simulink model "osss"  (R2024b)
settings: Solver=VariableStepAuto  StartTime=0.0  StopTime=100  RelTol=1e-3
values from neighbouring files (symbols this model uses):
  A4 = horzcat([0;0;0;0], A4)    [stabilita_AS.m]
  BB = [0; B]    [stabilita_AS.m]
settings Model: Creator=costa  LastModifiedBy=costa

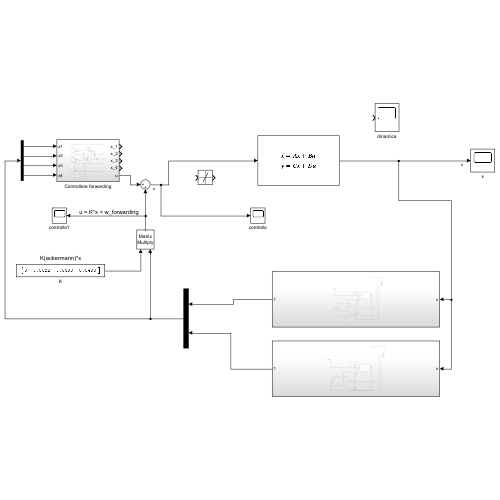
[thumbnail: Simulink's stored preview of the top-level diagram]
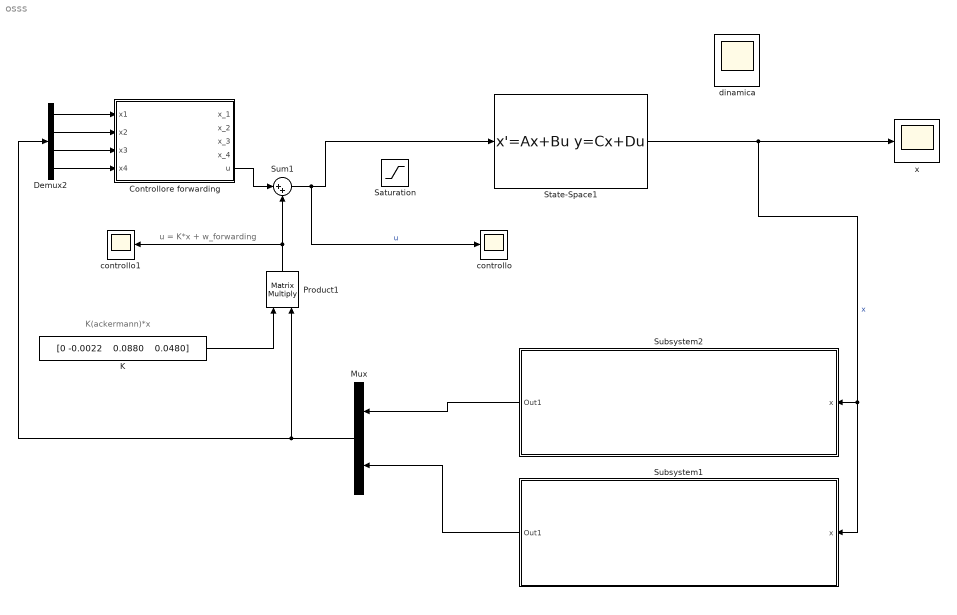
== system osss ==
  note: K(ackermann)*x
  note: u = K*x + w_forwarding
  Controllore forwarding : Subsystem
  Demux2 : Demux
  K : Constant  Value="[0 -0.0022    0.0880    0.0480]"  VectorParams1D=off
  Mux : Mux  Inputs=2
  Product1 : Product  Multiplication=Matrix(*)
  Saturation : Saturate
  State-Space1 : StateSpace  A=A4  B=BB  C=eye(4)  D=[0; 0; 0; 0]  InitialCondition=[1 1 1 1]
  Subsystem1 : Subsystem
  Subsystem2 : Subsystem
  Sum1 : Sum  Inputs=|++
  controllo : Scope
  controllo1 : Scope
  dinamica : Scope
  x : Scope
  wires:
  K/1 -> Product1/1
  Sum1/1 -> State-Space1/1, controllo/1  "u"
  Product1/1 -> controllo1/1, Sum1/2
  State-Space1/1 -> Subsystem2/1(x), Subsystem1/1(x), x/1  "x"
  Demux2/4 -> Controllore forwarding/4(x4)
  Demux2/3 -> Controllore forwarding/3(x3)
  Demux2/1 -> Controllore forwarding/1(x1)
  Demux2/2 -> Controllore forwarding/2(x2)
  Controllore forwarding/5(u) -> Sum1/1
  Mux/1 -> Demux2/1, Product1/2
  Subsystem1/1(Out1) -> Mux/2
  Subsystem2/1(Out1) -> Mux/1

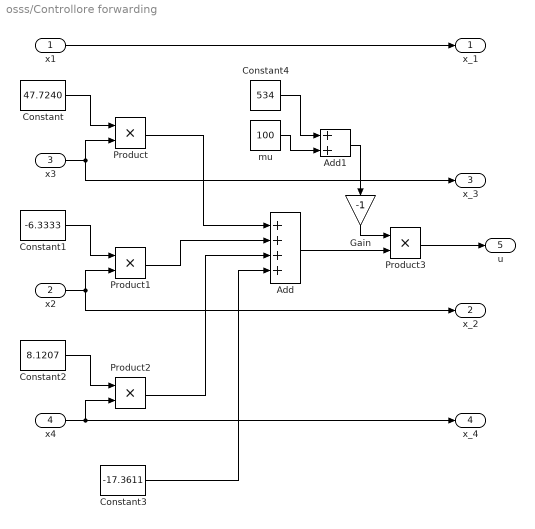
== system osss/Controllore forwarding ==
  x1 : Inport
  x2 : Inport  Port=2
  x3 : Inport  Port=3
  x4 : Inport  Port=4
  Add : Sum  Inputs=++++
  Add1 : Sum
  Constant : Constant  Value=47.7240
  Constant1 : Constant  Value=-6.3333
  Constant2 : Constant  Value=8.1207
  Constant3 : Constant  Value=-17.3611
  Constant4 : Constant  Value=534
  Gain : Gain  Gain=-1
  Product{,1..3} (4 alike) : Product
  mu : Constant  Value=100
  x_1 : Outport
  x_2 : Outport  Port=2
  x_3 : Outport  Port=3
  x_4 : Outport  Port=4
  u : Outport  Port=5
  wires:
  x3/1 -> x_3/1, Product/2
  Constant/1 -> Product/1
  Constant1/1 -> Product1/1
  x2/1 -> Product1/2, x_2/1
  Constant2/1 -> Product2/1
  x4/1 -> x_4/1, Product2/2
  Product/1 -> Add/1
  Product1/1 -> Add/2
  Product2/1 -> Add/3
  Constant3/1 -> Add/4
  Add/1 -> Product3/2
  Product3/1 -> u/1
  x1/1 -> x_1/1
  Constant4/1 -> Add1/1
  mu/1 -> Add1/2
  Add1/1 -> Gain/1
  Gain/1 -> Product3/1

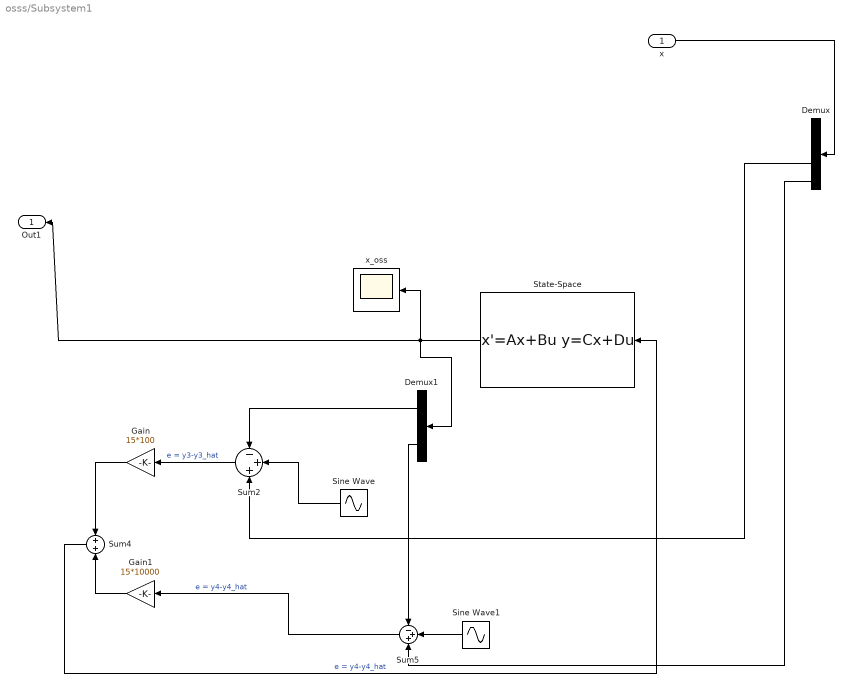
== system osss/Subsystem1 ==
  x : Inport
  Demux : Demux
  Demux1 : Demux  Outputs=2
  Gain : Gain  Gain=15*100
  Gain1 : Gain  Gain=15*10000
  Sine Wave : Sin  Amplitude=0.1  Frequency=2*pi*50  SampleTime=0
  Sine Wave1 : Sin  Amplitude=0.1  Frequency=2*pi*50  SampleTime=0
  State-Space : StateSpace  A=A4  B=BB  C=[0 0 1 0; 0 0 0 1]  D=[0; 0]  InitialCondition=[1 1 1 1]
  Sum2 : Sum  Inputs=-++
  Sum4 : Sum
  Sum5 : Sum  Inputs=-++
  x_oss : Scope
  Out1 : Outport
  wires:
  Gain1/1 -> Sum4/2
  State-Space/1 -> x_oss/1, Out1/1, Demux1/1
  x/1 -> Demux/1
  Sum5/1 -> Gain1/1  "e = y4-y4_hat"
  Sum2/1 -> Gain/1  "e = y3-y3_hat"
  Sine Wave1/1 -> Sum5/2
  Demux1/1 -> Sum2/1
  Demux/4 -> Sum5/3
  Sine Wave/1 -> Sum2/2
  Demux1/2 -> Sum5/1
  Sum4/1 -> State-Space/1  "e = y4-y4_hat"
  Demux/3 -> Sum2/3
  Gain/1 -> Sum4/1

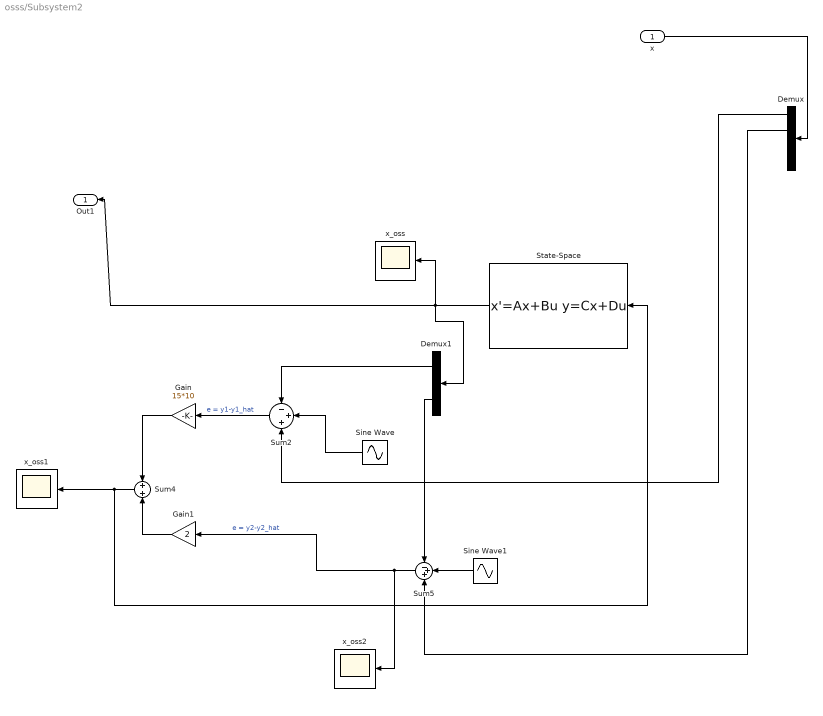
== system osss/Subsystem2 ==
  x : Inport
  Demux : Demux
  Demux1 : Demux  Outputs=2
  Gain : Gain  Gain=15*10
  Gain1 : Gain  Gain=2
  Sine Wave : Sin  Amplitude=0.1  Frequency=2*pi*50  SampleTime=0
  Sine Wave1 : Sin  Amplitude=0.1  Frequency=2*pi*50  SampleTime=0
  State-Space : StateSpace  A=A4  B=BB  C=[1 0 0 0; 0 1 0 0]  D=[0; 0]  InitialCondition=[0 0 0 0]  AbsoluteTolerance=1e-4
  Sum2 : Sum  Inputs=-++
  Sum4 : Sum
  Sum5 : Sum  Inputs=-++
  x_oss : Scope
  x_oss1 : Scope
  x_oss2 : Scope
  Out1 : Outport
  wires:
  Gain1/1 -> Sum4/2
  State-Space/1 -> x_oss/1, Out1/1, Demux1/1
  x/1 -> Demux/1
  Sum5/1 -> Gain1/1, x_oss2/1  "e = y2-y2_hat"
  Sum2/1 -> Gain/1  "e = y1-y1_hat"
  Sine Wave1/1 -> Sum5/2
  Demux1/1 -> Sum2/1
  Sine Wave/1 -> Sum2/2
  Demux1/2 -> Sum5/1
  Sum4/1 -> x_oss1/1, State-Space/1
  Gain/1 -> Sum4/1
  Demux/1 -> Sum2/3
  Demux/2 -> Sum5/3
